simulink model "Model"  (R2023b)
settings: Solver=ode4  StartTime=0.0  StopTime=7.121081656184960e+03  FixedStep=0.1  RelTol=1e-3
values from neighbouring files (symbols this model uses):
  astro_data = astronomicData    [main.m]
  in_cond = initialConditions(astro_data.n_eth)    [main.m]
  orbit_data = orbitData    [main.m]
  pert_data = perturbationData(orbit_data.n_sc)    [main.m]
  sc_data = spaceCraftData    [main.m]
undefined symbols (not defined in the file or in its folder): A_target, k1, k2, Kdx, Kdy, Kdz, Kpx, Kpy, Kpz, sensor_data
libraries: matrix_library x6, simulink x5, vrlib x4
(part 2 of 2)

== system Model/Complete model - KEEP COMMENTED/Spacecraft_Kinematics1/Orthonormalization ==
  note: $\text{The integration does not preserve the orthonormality of the matrix A, so an iterative method could be implemented. As the error is not high enough to impact substantially the solution, the orthonormalization method is applied only at the first iteration: }\\ A(t) = \frac{3}{2}A_0(t) - \frac{1}{2}A_0(t)A_0^T(t)A_0(t)\\ \text{Note also that this process can be applied only after a certain treshold as been reached to preserve computational power}$
  A_to_ortho : Inport
  Abs : Abs  SaturateOnIntegerOverflow=off
  Constant : Constant  Value=eye(3)
  Constant2 : Constant  Value=1e-6
  If : If  IfExpression=u1 ~= 9
  If Action Subsystem : Subsystem  TreatAsAtomicUnit=on
  If Action Subsystem1 : Subsystem  TreatAsAtomicUnit=on
  Less Than : RelationalOperator  Operator=<=  OutDataTypeStr=boolean  RndMeth=Simplest  InputSameDT=off
  Merge : Merge
  Product1 : Product  Inputs=**  Multiplication=Matrix(*)
  Subtract : Sum  Inputs=+-
  Sum of Elements : Sum  Inputs=+
  Transpose1 : Math  Operator=transpose
  A_ortho : Outport
  wires:
  [A_to_ortho] -> If Action Subsystem/1(A_to_ortho)
  [A_to_ortho] -> If Action Subsystem1/1(A_to_ortho)
  [A_to_ortho] -> Transpose1/1, Product1/1
  A_to_ortho/1 -> [A_to_ortho]
  Merge/1 -> A_ortho/1
  If Action Subsystem1/1(Out1) -> Merge/2
  If Action Subsystem/1(A_ortho) -> Merge/1
  If/2 -> If Action Subsystem1/Action
  If/1 -> If Action Subsystem/Action
  Sum of Elements/1 -> If/1
  Abs/1 -> Less Than/1
  Constant2/1 -> Less Than/2
  Constant/1 -> Subtract/2
  Less Than/1 -> Sum of Elements/1
  Transpose1/1 -> Product1/2
  Subtract/1 -> Abs/1
  Product1/1 -> Subtract/1

== system Model/Complete model - KEEP COMMENTED/Spacecraft_Kinematics1/omega_matrix ==
  note: $\text{Resulting matrix is:}\\ \matrix{0 & -\omega_3 & \omega_2 \cr \omega_3 & 0 & -\omega_1 \cr -\omega_2 & \omega_1 & 0}$
  omega : Inport
  Add : Sum  Inputs=+++
  Constant : Constant  Value=[0 0 0; 0 0 -1; 0 1 0]
  Constant1 : Constant  Value=[0 0 1; 0 0 0; -1 0 0]
  Constant2 : Constant  Value=[0 -1 0; 1 0 0; 0 0 0]
  Demux : Demux  Outputs=3
  Product : Product
  Product1 : Product
  Product2 : Product
  omega_matrix : Outport
  wires:
  Add/1 -> omega_matrix/1
  Product2/1 -> Add/3
  Product1/1 -> Add/2
  Product/1 -> Add/1
  Demux/3 -> Product2/1
  Constant2/1 -> Product2/2
  Constant1/1 -> Product1/2
  Demux/2 -> Product1/1
  Demux/1 -> Product/2
  Constant/1 -> Product/1
  omega/1 -> Demux/1

== system Model/Complete model - KEEP COMMENTED/r_integration/Subsystem ==
  Vector : Inport  OutDataTypeStr=double
  Dot Product : DotProduct  OutDataTypeStr=Inherit: Inherit via internal rule
  Sqrt : Sqrt
  Norm : Outport  OutDataTypeStr=double
  wires:
  Dot Product/1 -> Sqrt/1
  Vector/1 -> Dot Product/2, Dot Product/1
  Sqrt/1 -> Norm/1

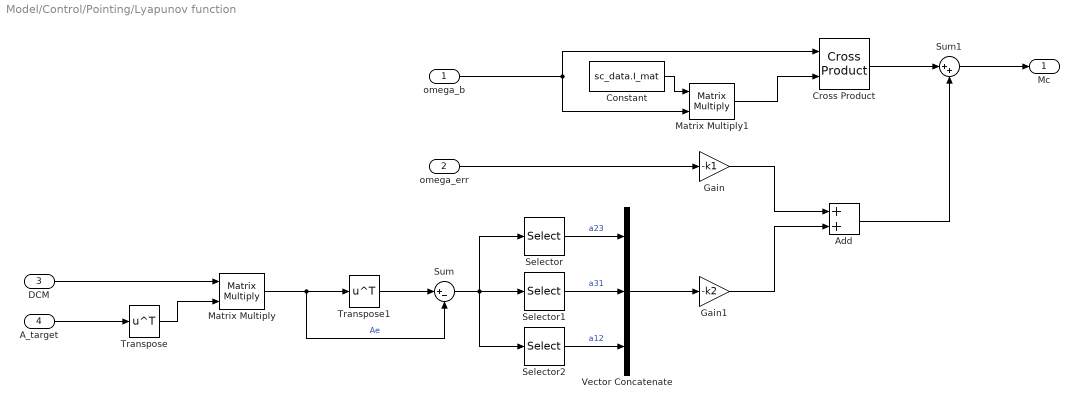
== system Model/Control/Pointing/Lyapunov function ==
  omega_b : Inport
  omega_err : Inport  Port=2
  DCM : Inport  Port=3
  A_target : Inport  Port=4
  Add : Sum
  Constant : Constant  Value=sc_data.I_mat
  Cross Product : matrix_library/Cross Product
  Gain : Gain  Gain=-k1
  Gain1 : Gain  Gain=-k2
  Matrix Multiply : Product  Multiplication=Matrix(*)
  Matrix Multiply1 : Product  Multiplication=Matrix(*)
  Selector : Selector  NumberOfDimensions=2  InputPortWidth=3  IndexOptions=Index vector (dialog),Index vector (dialog)  Indices=2,3  OutputSizes=1,1
  Selector1 : Selector  NumberOfDimensions=2  InputPortWidth=3  IndexOptions=Index vector (dialog),Index vector (dialog)  Indices=3,1  OutputSizes=1,1
  Selector2 : Selector  NumberOfDimensions=2  InputPortWidth=3  IndexOptions=Index vector (dialog),Index vector (dialog)  Indices=1,2  OutputSizes=1,1
  Sum : Sum  Inputs=|+-
  Sum1 : Sum  Inputs=|++
  Transpose : Math  Operator=transpose
  Transpose1 : Math  Operator=transpose
  Vector Concatenate : Concatenate  NumInputs=3
  Mc : Outport
  wires:
  omega_err/1 -> Gain/1
  Sum1/1 -> Mc/1
  Gain/1 -> Add/1
  DCM/1 -> Matrix Multiply/1
  A_target/1 -> Transpose/1
  Transpose/1 -> Matrix Multiply/2
  Matrix Multiply/1 -> Sum/2, Transpose1/1  "Ae"
  Transpose1/1 -> Sum/1
  Sum/1 -> Selector2/1, Selector/1, Selector1/1
  Selector/1 -> Vector Concatenate/1  "a23"
  Selector1/1 -> Vector Concatenate/2  "a31"
  Selector2/1 -> Vector Concatenate/3  "a12"
  Vector Concatenate/1 -> Gain1/1
  Gain1/1 -> Add/2
  Add/1 -> Sum1/2
  Cross Product/1 -> Sum1/1
  Matrix Multiply1/1 -> Cross Product/2
  Constant/1 -> Matrix Multiply1/1
  omega_b/1 -> Matrix Multiply1/2, Cross Product/1

== system Model/Perturbations/GG_perturbation/Subsystem ==
  Inertia matrix : Inport
  c1 c2 c3 : Inport  Port=2
  Inverse Inertia : Inport  Port=3
  Cross Product : matrix_library/Cross Product
  Matrix Divide : Product  Inputs=**  Multiplication=Matrix(*)
  Product : Product  Multiplication=Matrix(*)
  Reshape : Reshape  OutputDimensionality=Column vector (2-D)
  Reshape1 : Reshape  OutputDimensionality=Row vector (2-D)
  M_GG_vec : Outport
  wires:
  Matrix Divide/1 -> Reshape1/1
  Inertia matrix/1 -> Product/1  "I_matrix"
  Product/1 -> Cross Product/1
  Inverse Inertia/1 -> Matrix Divide/1
  c1 c2 c3/1 -> Reshape/1
  Cross Product/1 -> Matrix Divide/2
  Reshape/1 -> Cross Product/2, Product/2  "[c1 c2 c3]"
  Reshape1/1 -> M_GG_vec/1  "[c1 c2 c3]"

== system Model/Perturbations/Magnetic/Apply_inertia ==
  M : Inport
  Constant : Constant  Value=sc_data.I_inv
  Matrix Multiply : Product  Multiplication=Matrix(*)
  Reshape : Reshape  OutputDimensionality=Column vector (2-D)
  Reshape1 : Reshape  OutputDimensionality=Row vector (2-D)
  Torque_omega_dot : Outport
  wires:
  M/1 -> Reshape/1
  Matrix Multiply/1 -> Reshape1/1
  Reshape/1 -> Matrix Multiply/2
  Reshape1/1 -> Torque_omega_dot/1
  Constant/1 -> Matrix Multiply/1

== system Model/Perturbations/SRP/Apply_inertia ==
  M : Inport
  Constant : Constant  Value=sc_data.I_inv
  Matrix Multiply : Product  Multiplication=Matrix(*)
  Reshape : Reshape  OutputDimensionality=Column vector (2-D)
  Reshape1 : Reshape  OutputDimensionality=Row vector (2-D)
  Torque_omega_dot : Outport
  wires:
  M/1 -> Reshape/1
  Matrix Multiply/1 -> Reshape1/1
  Reshape/1 -> Matrix Multiply/2
  Reshape1/1 -> Torque_omega_dot/1
  Constant/1 -> Matrix Multiply/1

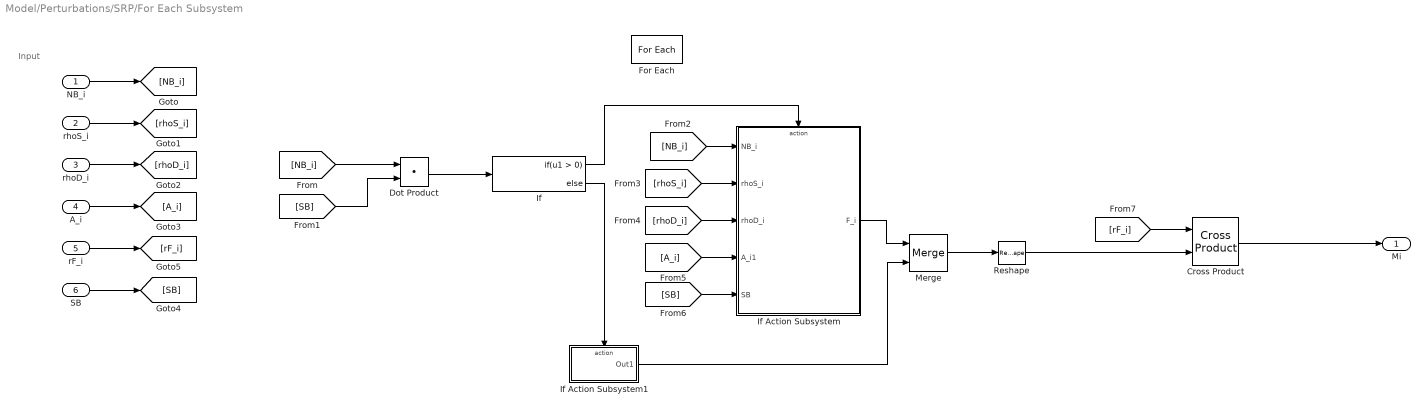
== system Model/Perturbations/SRP/For Each Subsystem ==
  note: Input
  NB_i : Inport  Partition=on  PartitionDimension=1  PartitionWidth=1  PartitionOffset=0
  rhoS_i : Inport  Port=2  Partition=on  PartitionDimension=1  PartitionWidth=1  PartitionOffset=0
  rhoD_i : Inport  Port=3  Partition=on  PartitionDimension=1  PartitionWidth=1  PartitionOffset=0
  A_i : Inport  Port=4  Partition=on  PartitionDimension=1  PartitionWidth=1  PartitionOffset=0
  rF_i : Inport  Port=5  Partition=on  PartitionDimension=1  PartitionWidth=1  PartitionOffset=0
  SB : Inport  Port=6
  Cross Product : matrix_library/Cross Product
  Dot Product : DotProduct  OutDataTypeStr=Inherit: Inherit via internal rule
  For Each : ForEach  DisableCoverage=on
  If : If
  If Action Subsystem : Subsystem  TreatAsAtomicUnit=on
  If Action Subsystem1 : Subsystem  TreatAsAtomicUnit=on
  Merge : Merge
  Reshape : Reshape  OutputDimensionality=Row vector (2-D)
  Mi : Outport  ConcatenationDimension=1
  wires:
  NB_i/1 -> [NB_i]
  rhoS_i/1 -> [rhoS_i]
  rhoD_i/1 -> [rhoD_i]
  A_i/1 -> [A_i]
  SB/1 -> [SB]
  [NB_i] -> Dot Product/1
  [SB] -> Dot Product/2
  Dot Product/1 -> If/1
  If/1 -> If Action Subsystem/Action
  If/2 -> If Action Subsystem1/Action
  Merge/1 -> Reshape/1
  If Action Subsystem1/1(Out1) -> Merge/2
  If Action Subsystem/1(F_i) -> Merge/1
  [NB_i] -> If Action Subsystem/1(NB_i)
  [rhoS_i] -> If Action Subsystem/2(rhoS_i)
  [rhoD_i] -> If Action Subsystem/3(rhoD_i)
  [A_i] -> If Action Subsystem/4(A_i1)
  [SB] -> If Action Subsystem/5(SB)
  Reshape/1 -> Cross Product/2
  Cross Product/1 -> Mi/1
  rF_i/1 -> [rF_i]
  [rF_i] -> Cross Product/1

== system Model/Perturbations/SRP/Norm ==
  In1 : Inport
  Dot Product : DotProduct  OutDataTypeStr=Inherit: Inherit via internal rule
  Sqrt : Sqrt
  Out1 : Outport
  wires:
  In1/1 -> Dot Product/1, Dot Product/2
  Dot Product/1 -> Sqrt/1
  Sqrt/1 -> Out1/1

== system Model/Complete model - KEEP COMMENTED/Spacecraft_Kinematics1/Orthonormalization/If Action Subsystem ==
  A_to_ortho : Inport
  Action Port : ActionPort
  Add : Sum  Inputs=+-
  Gain : Gain  Gain=3/2
  Gain1 : Gain  Gain=1/2
  Product : Product  Inputs=***  Multiplication=Matrix(*)
  Transpose : Math  Operator=transpose
  A_ortho : Outport
  wires:
  Add/1 -> A_ortho/1
  Product/1 -> Gain1/1
  A_to_ortho/1 -> Gain/1, Product/1, Transpose/1, Product/3
  Transpose/1 -> Product/2
  Gain1/1 -> Add/2
  Gain/1 -> Add/1

== system Model/Complete model - KEEP COMMENTED/Spacecraft_Kinematics1/Orthonormalization/If Action Subsystem1 ==
  A_to_ortho : Inport
  Action Port : ActionPort
  Out1 : Outport
  wires:
  A_to_ortho/1 -> Out1/1

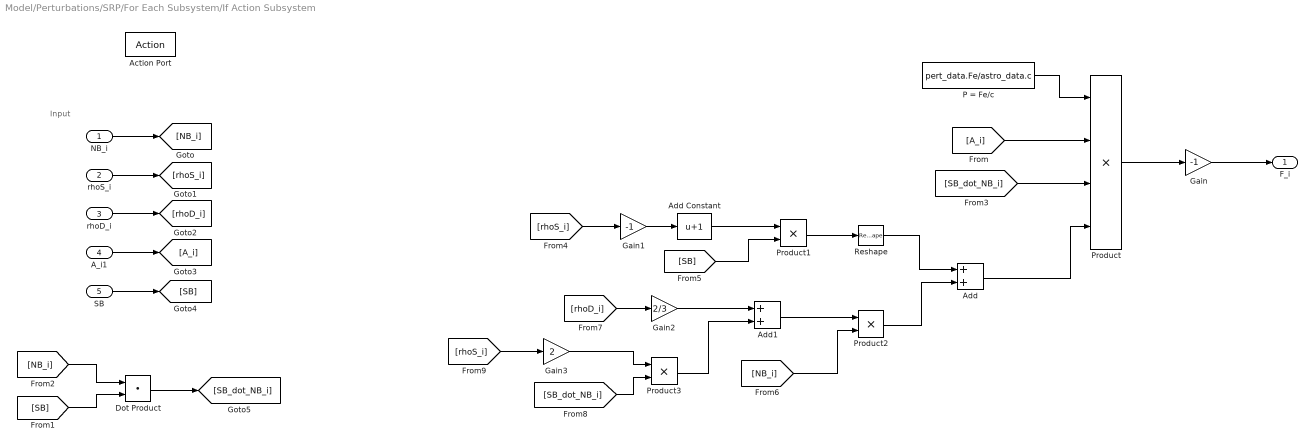
== system Model/Perturbations/SRP/For Each Subsystem/If Action Subsystem ==
  note: Input
  NB_i : Inport
  rhoS_i : Inport  Port=2
  rhoD_i : Inport  Port=3
  A_i1 : Inport  Port=4
  SB : Inport  Port=5
  Action Port : ActionPort  ActionPortLabel=if(u1 > 0)
  Add : Sum
  Add Constant : Bias  Bias=1  SaturateOnIntegerOverflow=off
  Add1 : Sum
  Dot Product : DotProduct  OutDataTypeStr=Inherit: Inherit via internal rule
  Gain : Gain  Gain=-1
  Gain1 : Gain  Gain=-1
  Gain2 : Gain  Gain=2/3
  Gain3 : Gain  Gain=2
  P = Fe/c : Constant  Value=pert_data.Fe/astro_data.c
  Product : Product  Inputs=4
  Product1 : Product
  Product2 : Product
  Product3 : Product
  Reshape : Reshape  OutputDimensionality=Row vector (2-D)
  F_i : Outport
  wires:
  Product/1 -> Gain/1
  Gain/1 -> F_i/1
  P = Fe/c/1 -> Product/1
  [A_i] -> Product/2
  A_i1/1 -> [A_i]
  rhoS_i/1 -> [rhoS_i]
  SB/1 -> [SB]
  NB_i/1 -> [NB_i]
  rhoD_i/1 -> [rhoD_i]
  [NB_i] -> Dot Product/1
  [SB] -> Dot Product/2
  Dot Product/1 -> [SB_dot_NB_i]
  [SB_dot_NB_i] -> Product/3
  Add/1 -> Product/4
  [rhoS_i] -> Gain1/1
  Gain1/1 -> Add Constant/1
  Add Constant/1 -> Product1/1
  [SB] -> Product1/2
  Product1/1 -> Reshape/1
  Product2/1 -> Add/2
  [NB_i] -> Product2/2
  Add1/1 -> Product2/1
  [rhoD_i] -> Gain2/1
  Gain2/1 -> Add1/1
  Product3/1 -> Add1/2
  [SB_dot_NB_i] -> Product3/2
  [rhoS_i] -> Gain3/1
  Gain3/1 -> Product3/1
  Reshape/1 -> Add/1

== system Model/Perturbations/SRP/For Each Subsystem/If Action Subsystem1 ==
  Action Port : ActionPort  ActionPortLabel=else
  Constant : Constant  Value=zeros(1,3)
  Out1 : Outport
  wires:
  Constant/1 -> Out1/1

== matlab function Model/Subsystem/MATLAB Function ==
  data: u input; y output
function y = fcn(u)

y = det(u);

== matlab function Model/Subsystem/MATLAB Function2 ==
  data: u input; y output
function y = fcn(u)

vals = u(isfinite(u));

y = mean(vals, 'all');

== matlab function Model/Subsystem/MATLAB Function1 ==
  data: u input; y output
function y = fcn(u)

y = mean(u, 'all');
